simulink model "Optimizador_Programacion_Lineal"  (R2017a)
settings: Solver=ode4  StartTime=0.0  StopTime=10.0  FixedStep=1e-6  MaxStep=1e-4  RelTol=1e-3
InitFcn:
  | SimulinkInit
settings Model: Creator=Administrador  LastModifiedBy=Administrador
settings OptimizationCC: DefaultParameterBehavior=Inlined  PassReuseOutputArgsAs=Individual arguments
settings DebuggingCC: ParameterTunabilityLossMsg=error
settings SFSimCC: MATLABDynamicMemAlloc=off
settings RTWCC: SystemTargetFile=ert.tlc  TemplateMakefile=ert_default_tmf  Description=Embedded Coder  GenerateReport=on  IncludeHyperlinkInReport=on  LaunchReport=on  GenerateTraceInfo=on  GenerateTraceReport=on  GenerateTraceReportSl=on  GenerateTraceReportSf=on  GenerateTraceReportEml=on
settings CodeAppCC: ForceParamTrailComments=on  IgnoreCustomStorageClasses=off  OperatorAnnotations=on  SimulinkDataObjDesc=on  SFDataObjDesc=on  MATLABFcnDesc=on  InsertBlockDesc=on  MATLABSourceComments=on
settings ERTTargetCC: TargetLangStandard=C99 (ISO)  GenerateSampleERTMain=on  SupportContinuousTime=on  SupportNonInlinedSFcns=on  SupportVariableSizeSignals=on  InlinedParameterPlacement=NonHierarchical  ERTCustomFileTemplate=example_file_process.tlc

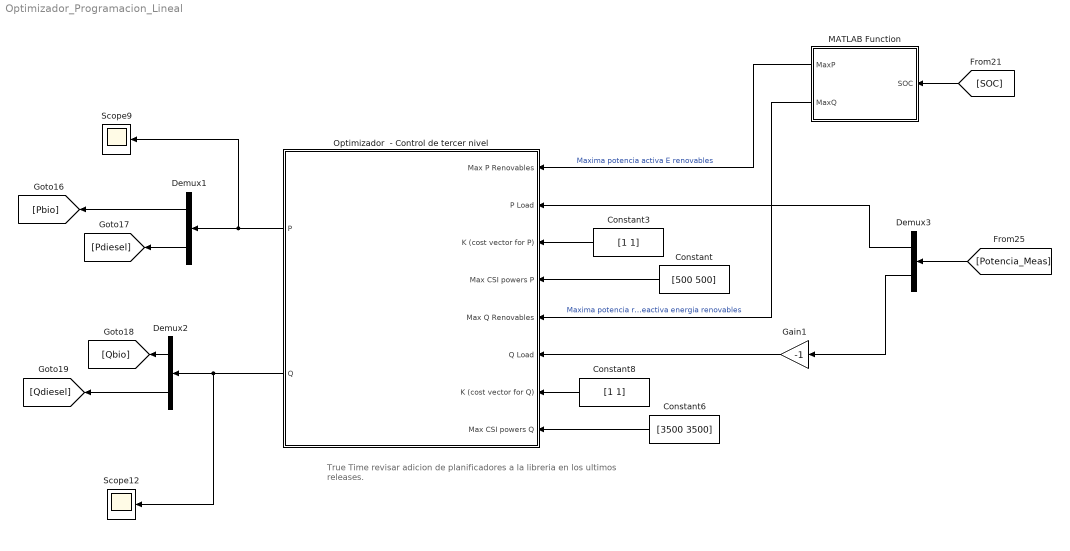
== system Optimizador_Programacion_Lineal ==
  note: True Time revisar adicion de planificadores
      | a la libreria en los ultimos releases.
  Constant : Constant  Value=[500 500]
  Constant3 : Constant  Value=[1 1]
  Constant6 : Constant  Value=[3500 3500]
  Constant8 : Constant  Value=[1 1]
  Demux1 : Demux  Outputs=2
  Demux2 : Demux  Outputs=2
  Demux3 : Demux  Outputs=2
  Gain1 : Gain  Gain=-1
  MATLAB Function : MATLAB Function  TreatAsAtomicUnit=on
  Optimizador  - Control de tercer nivel : Subsystem
  Scope12 : Scope
  Scope9 : Scope
  wires:
  Constant/1 -> Optimizador  - Control de tercer nivel/4(Max CSI powers P)
  MATLAB Function/2(MaxQ) -> Optimizador  - Control de tercer nivel/5(Max Q Renovables)  "Maxima potencia reactiva energia renovables"
  [Potencia_Meas] -> Demux3/1
  Demux3/1 -> Optimizador  - Control de tercer nivel/2(P Load)
  Constant6/1 -> Optimizador  - Control de tercer nivel/8(Max CSI powers Q)
  Constant3/1 -> Optimizador  - Control de tercer nivel/3(K (cost vector for P))
  Optimizador  - Control de tercer nivel/1(P) -> Demux1/1, Scope9/1
  Constant8/1 -> Optimizador  - Control de tercer nivel/7(K (cost vector for Q))
  MATLAB Function/1(MaxP) -> Optimizador  - Control de tercer nivel/1(Max P Renovables)  "Maxima potencia activa E renovables"
  [SOC] -> MATLAB Function/1(SOC)
  Optimizador  - Control de tercer nivel/2(Q) -> Demux2/1, Scope12/1
  Demux2/2 -> [Qdiesel]
  Demux2/1 -> [Qbio]
  Demux3/2 -> Gain1/1
  Demux1/1 -> [Pbio]
  Demux1/2 -> [Pdiesel]
  Gain1/1 -> Optimizador  - Control de tercer nivel/6(Q Load)

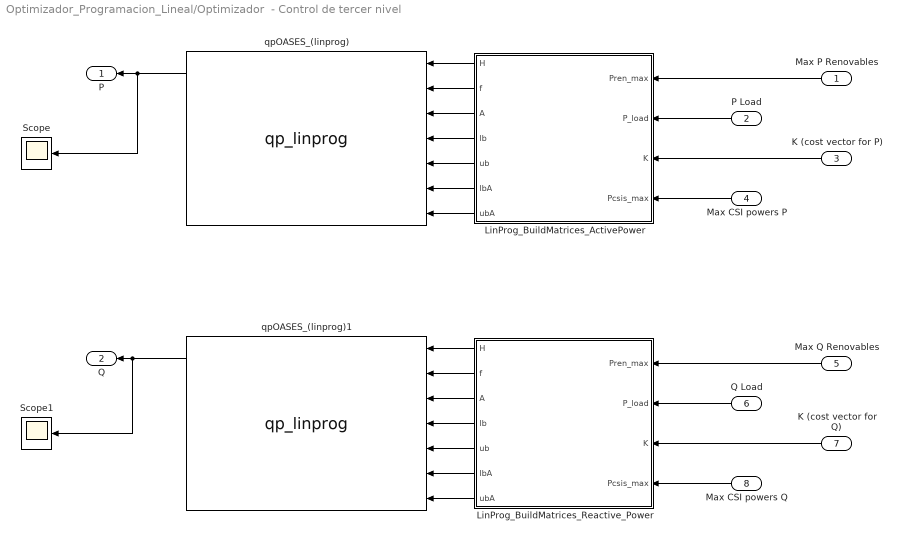
== system Optimizador_Programacion_Lineal/Optimizador  - Control de tercer nivel ==
  Max P Renovables : Inport
  P Load : Inport  Port=2
  K (cost vector for P) : Inport  Port=3
  Max CSI powers P : Inport  Port=4
  Max Q Renovables : Inport  Port=5
  Q Load : Inport  Port=6
  K (cost vector for Q) : Inport  Port=7
  Max CSI powers Q : Inport  Port=8
  LinProg_BuildMatrices_ActivePower : MATLAB Function  TreatAsAtomicUnit=on
  LinProg_BuildMatrices_Reactive_Power : MATLAB Function  TreatAsAtomicUnit=on
  Scope : Scope
  Scope1 : Scope
  qpOASES_(linprog) : S-Function  FunctionName=qp_linprog  SFunctionDeploymentMode=off  EnableBusSupport=off
  qpOASES_(linprog)1 : S-Function  FunctionName=qp_linprog  SFunctionDeploymentMode=off  EnableBusSupport=off
  P : Outport
  Q : Outport  Port=2
  wires:
  Max CSI powers P/1 -> LinProg_BuildMatrices_ActivePower/4(Pcsis_max)
  Max P Renovables/1 -> LinProg_BuildMatrices_ActivePower/1(Pren_max)
  LinProg_BuildMatrices_ActivePower/6(lbA) -> qpOASES_(linprog)/6
  LinProg_BuildMatrices_ActivePower/5(ub) -> qpOASES_(linprog)/5
  LinProg_BuildMatrices_ActivePower/7(ubA) -> qpOASES_(linprog)/7
  LinProg_BuildMatrices_ActivePower/2(f) -> qpOASES_(linprog)/2
  LinProg_BuildMatrices_ActivePower/4(lb) -> qpOASES_(linprog)/4
  LinProg_BuildMatrices_ActivePower/1(H) -> qpOASES_(linprog)/1
  K (cost vector for P)/1 -> LinProg_BuildMatrices_ActivePower/3(K)
  P Load/1 -> LinProg_BuildMatrices_ActivePower/2(P_load)
  LinProg_BuildMatrices_ActivePower/3(A) -> qpOASES_(linprog)/3
  LinProg_BuildMatrices_Reactive_Power/1(H) -> qpOASES_(linprog)1/1
  LinProg_BuildMatrices_Reactive_Power/5(ub) -> qpOASES_(linprog)1/5
  LinProg_BuildMatrices_Reactive_Power/3(A) -> qpOASES_(linprog)1/3
  LinProg_BuildMatrices_Reactive_Power/4(lb) -> qpOASES_(linprog)1/4
  LinProg_BuildMatrices_Reactive_Power/6(lbA) -> qpOASES_(linprog)1/6
  LinProg_BuildMatrices_Reactive_Power/2(f) -> qpOASES_(linprog)1/2
  LinProg_BuildMatrices_Reactive_Power/7(ubA) -> qpOASES_(linprog)1/7
  qpOASES_(linprog)/1 -> Scope/1, P/1
  qpOASES_(linprog)1/1 -> Scope1/1, Q/1
  Q Load/1 -> LinProg_BuildMatrices_Reactive_Power/2(P_load)
  K (cost vector for Q)/1 -> LinProg_BuildMatrices_Reactive_Power/3(K)
  Max Q Renovables/1 -> LinProg_BuildMatrices_Reactive_Power/1(Pren_max)
  Max CSI powers Q/1 -> LinProg_BuildMatrices_Reactive_Power/4(Pcsis_max)

== matlab function Optimizador_Programacion_Lineal/MATLAB Function ==
  data: SOC input; MaxP output; MaxQ output
function [MaxP, MaxQ] = fcn(SOC)


%  funcion que calcula la potencia maxima que puede suministrar las fuentes
%  renovables deacuerdo a la cantidad de carga que hay almancenada en la
%  bateria. esta va de 0 a 100%


% estoc valores que aparecen a continuacion se pusieron de manera
% arbitraria. corresponde a una persona con especialidad en la parte de
% potencia electrica determinar el verdadero algoritmo para hallar la
% potencia que deberia suministrar el nodo de energia renovable deacuerdo a
% la carga de la bateria.

MaxP = 0;
MaxQ = 0;

if( SOC >= 90 )
    MaxP = 500;
    MaxQ = 5000;
end

if( SOC <= 90 )
    MaxP = 200;
    MaxQ = 4000;
end

if( SOC <= 70 )
    MaxP = 100;
    MaxQ = 1000;
end

if( SOC <= 60 )
    MaxP = 50;
    MaxQ = 500;
end

== matlab function Optimizador_Programacion_Lineal/Optimizador  - Control de tercer nivel/LinProg_BuildMatrices_ActivePower ==
  data: H output; Pren_max input; f output; P_load input; K input; A output; lb output; ub output; lbA output; ubA output; Pcsis_max input
function [H, f, A, lb, ub, lbA, ubA] = fcn(Pren_max, P_load, K, Pcsis_max)

% Pr_max es la potencia maxima que puede suministrar el nodo de energias
% renovables.

% P_load es la potencia que consume la carga. ambas potencias son un vector
% de 2 componentes donde la primera componenete es la potencia activa y la
% segunda componenete es la potencia reactiva.

% Kp y Kq corresponde a un vector con los costos de la energia activa y 
% reactiva respectivamente para cada uno de los convertidores, en este caso
% bio y diesel solamente pero pueden agregarse tantas fuentes como se
% desee.

% Pin_max Qin_max corresponde a un vector con los valores maximos de
% potencia activa y reactiva que pueden generar cada una de las otras 
% fuentes diferentes a energias alternativas.


% El bloque qpOASES_(linprog) es un bloque que resuelve el problema standar
% de optimizacion cuadratica :
% 1/2 x' H x + x' f
% sujeto a unas restricciones. la matriz H corresponde a la parte
% cuadratica del problema mientras que f corresponde a la parte lineal. es
% decir que haciendo H = matriz de zeros, es posible reutilizar el bloque
% para solucionar problemas de programacion lineal, que es justamente lo
% que se hace en esta parte del modelo.

% La presente matlab function tiene como tarea formar las matrices f
% y A de restricciones apropiadas para que el bloque de qp oases realice la
% funcione de programacion lineal.

Pm = sum(Pcsis_max); % potencia activa maxima que pueden entregar todas las fuentes (en este caso bio y diesel)


D = P_load - Pren_max; % diferencia entre la potencia que puede generar
% renovables con la que consume la carga.


     % % % % % % % % % % % % % % % % % % % % % % % % % % % % %  
    % Formacion de las entradas para la programacion lineal.  %
     % % % % % % % % % % % % % % % % % % % % % % % % % % % % %  
     
% parte cuadratica de la funcion de coste que se pone en zeros para
% transformarlo en un problema de programacion lineal.
H = zeros(1, length(K)^2);

% funcion de coste lineal.
f = K;

% matriz de restricciones.
% esta formada con la idea de definir que la suma de todas las potencias
% deben almenos cubrir la cantidad de energia activa y reactiva que no
% puede suministrar renovables.
A = ones(1, length(K));

lb = zeros(1, length(K)); % potencia minima que puede generar cada uno de los generadores.
ub = [Pcsis_max]; % potencia maxima que pueden generar cada uno de los generadores.

ubA = [Pm]; % tambien esta relacionado con la potencia min, es un
% requerimiento para el blque de programacion lineal.

% depenediendo la diferencia entre la potencia que pide la carga y la que
% pueden suministrar energias renovables entonces lbA debe establecerce de
% manera conveniente para que el problema de programacion lineal tenga
% solucion.

% restriccion limite inferior para la potencia activa
if(D > 0) % en caso de que renovables no baste para alimentar la carga...
    if(D >= Pm)
        vp = Pm;
    else
        vp = D(1);
    end
else % si renovables basta para alimentar la carga. es decir D = 0 ó negativo
    vp = 0;
end

lbA = vp;

== matlab function Optimizador_Programacion_Lineal/Optimizador  - Control de tercer nivel/LinProg_BuildMatrices_Reactive_Power ==
  data: H output; Pren_max input; f output; P_load input; K input; A output; lb output; ub output; lbA output; ubA output; Pcsis_max input
function [H, f, A, lb, ub, lbA, ubA] = fcn(Pren_max, P_load, K, Pcsis_max)

% Pr_max es la potencia maxima que puede suministrar el nodo de energias
% renovables.

% P_load es la potencia que consume la carga. ambas potencias son un vector
% de 2 componentes donde la primera componenete es la potencia activa y la
% segunda componenete es la potencia reactiva.

% Kp y Kq corresponde a un vector con los costos de la energia activa y 
% reactiva respectivamente para cada uno de los convertidores, en este caso
% bio y diesel solamente pero pueden agregarse tantas fuentes como se
% desee.

% Pin_max Qin_max corresponde a un vector con los valores maximos de
% potencia activa y reactiva que pueden generar cada una de las otras 
% fuentes diferentes a energias alternativas.


% El bloque qpOASES_(linprog) es un bloque que resuelve el problema standar
% de optimizacion cuadratica :
% 1/2 x' H x + x' f
% sujeto a unas restricciones. la matriz H corresponde a la parte
% cuadratica del problema mientras que f corresponde a la parte lineal. es
% decir que haciendo H = matriz de zeros, es posible reutilizar el bloque
% para solucionar problemas de programacion lineal, que es justamente lo
% que se hace en esta parte del modelo.

% La presente matlab function tiene como tarea formar las matrices f
% y A de restricciones apropiadas para que el bloque de qp oases realice la
% funcione de programacion lineal.

Pm = sum(Pcsis_max); % potencia activa maxima que pueden entregar todas las fuentes (en este caso bio y diesel)


D = P_load - Pren_max; % diferencia entre la potencia que puede generar
% renovables con la que consume la carga.


     % % % % % % % % % % % % % % % % % % % % % % % % % % % % %  
    % Formacion de las entradas para la programacion lineal.  %
     % % % % % % % % % % % % % % % % % % % % % % % % % % % % %  
     
% parte cuadratica de la funcion de coste que se pone en zeros para
% transformarlo en un problema de programacion lineal.
H = zeros(1, length(K)^2);

% funcion de coste lineal.
f = K;

% matriz de restricciones.
% esta formada con la idea de definir que la suma de todas las potencias
% deben almenos cubrir la cantidad de energia activa y reactiva que no
% puede suministrar renovables.
A = ones(1, length(K));

lb = zeros(1, length(K)); % potencia minima que puede generar cada uno de los generadores.
ub = [Pcsis_max]; % potencia maxima que pueden generar cada uno de los generadores.

ubA = [Pm]; % tambien esta relacionado con la potencia min, es un
% requerimiento para el blque de programacion lineal.

% depenediendo la diferencia entre la potencia que pide la carga y la que
% pueden suministrar energias renovables entonces lbA debe establecerce de
% manera conveniente para que el problema de programacion lineal tenga
% solucion.

% restriccion limite inferior para la potencia activa
if(D > 0) % en caso de que renovables no baste para alimentar la carga...
    if(D >= Pm)
        vp = Pm;
    else
        vp = D(1);
    end
else % si renovables basta para alimentar la carga. es decir D = 0 ó negativo
    vp = 0;
end

lbA = vp;
